simulink model "BMD_2_backup"  (R2025b)
settings: Solver=FixedStepAuto  StartTime=0.0  StopTime=15  FixedStep=0.005  RelTol=1e-3
values from neighbouring files (symbols this model uses):
  FPV_mass = 0.8    [Soft.m]
  g = 9.81    [Soft.m]
  ks = 0    [Soft.m]
  p_0 = 1013.25    [Soft.m]
  Q2Ts = forcetomotors()    [Soft.m]    (also in forcetomotors.m = inv(Ts2Q))
  takeOffDuration = 2    [Soft.m]
  Ts = 0.005    [Soft.m]
undefined symbols (not defined in the file or in its folder): CdA, DiscIntNeverNeededParam, Dw, kd_dz, kd_pos_dx, kd_pos_dy, kd_pq, kd_pr, kd_y, kd_z, ki_dz, ki_pos_dx, ki_pos_dy, ki_pq, ki_pr, ki_y, ki_z, kp_dz, kp_pos_dx, kp_pos_dy, kp_pos_x, kp_pos_y, kp_pq, kp_pr, kp_y, kp_z, pInitialization, rho
libraries: simulink x43, discretizing x18, slpidlib x3, SignalEditorBlockLib x2, shared6dof x1, dynamicsLibrary x1, aerolibasang x1, aerolibnav x1
(part 8 of 22)

== system BMD_2_backup/FCS/filters/Subsystem1/pitch_kalman ==
  ax,ay,az : Inport
  pitch : Inport  Port=2
  Atan2 : Trigonometry  Operator=atan2
  Compare To Constant : simulink/Logic and Bit Operations/Compare To Constant  relop=<=  const=8.5  OutDataTypeStr=boolean
  Compare To Constant1 : simulink/Logic and Bit Operations/Compare To Constant  relop=>=  const=11.5  OutDataTypeStr=boolean
  Data Type Conversion3 : DataTypeConversion  OutDataTypeStr=single  SaturateOnIntegerOverflow=off  RndMeth=Floor
  Demux : Demux  Outputs=3
  Gain1 : Gain  Gain=-1
  Kalman Filter1 : Subsystem  AncestorBlock=cstblocks/State Estimation/Kalman Filter  mask(ctrlKalmanFilter){TimeDomain=Discrete-Time, UseCurrentEstimator=on, ModelSource=Individual A, B, C, D matrices, ModelSourceVariable=ss(0.95,1,1,0,1), A=[1 -Ts;0 1], B=[Ts;0], C=[1 0], D=0, NumberOfStates=1, NumberOfInputs=1, NumberOfOutputs=1, InitialEstimateSource=Dialog, X0=[0; 0], P0=10, UseK=off, UseGH=off, NumberOfProcessNoiseInputs=1, G=1, TimeInvariantG=on, H=0, TimeInvariantH=on, Q=[0.001 0; 0 0.003], TimeInvariantQ=on, R=[1.0], TimeInvariantR=on, N=0, TimeInvariantN=on, AddInputPort=on, AddEnablePort=off, ExternalReset=None, OutputEstimatedY=off, OutputP=off, Ts=Ts}
      mask prompts: TimeDomain "Controllib:blocks:maskPromptKFTimeDomain"; UseCurrentEstimator "Controllib:blocks:maskPromptKFUseCurrentMeasurement"; ModelSource "Controllib:blocks:maskPromptKFModelSource"; ModelSourceVariable "Controllib:blocks:maskPromptKFModelSourceVariable"; A "Controllib:blocks:maskPromptKFA"; B "Controllib:blocks:maskPromptKFB"; C "Controllib:blocks:maskPromptKFC"; D "Controllib:blocks:maskPromptKFD"; NumberOfStates "Controllib:blocks:maskPromptKFNumberOfStates"; NumberOfInputs "Controllib:blocks:maskPromptKFNumberOfInputs"; NumberOfOutputs "Controllib:blocks:maskPromptKFNumberOfOutputs"; InitialEstimateSource "Controllib:blocks:maskPromptKFSource"; X0 "Controllib:blocks:maskPromptKFX0DT"; P0 "Controllib:blocks:maskPromptKFP0DT"; UseK "Controllib:blocks:maskPromptKFUseK"; UseGH "Controllib:blocks:maskPromptKFUseGH"; NumberOfProcessNoiseInputs "Controllib:blocks:maskPromptKFNumberOfProcessNoiseInputs"; G "Controllib:blocks:maskPromptKFG"; TimeInvariantG "Controllib:blocks:maskPromptKFTimeInvariantG"; H "Controllib:blocks:maskPromptKFH"; TimeInvariantH "Controllib:blocks:maskPromptKFTimeInvariantH"; Q "Controllib:blocks:maskPromptKFQ"; TimeInvariantQ "Controllib:blocks:maskPromptKFTimeInvariantQ"; R "Controllib:blocks:maskPromptKFR"; TimeInvariantR "Controllib:blocks:maskPromptKFTimeInvariantR"; N "Controllib:blocks:maskPromptKFN"; TimeInvariantN "Controllib:blocks:maskPromptKFTimeInvariantN"; AddInputPort "Controllib:blocks:maskPromptKFAddInputPort"; AddEnablePort "Controllib:blocks:maskPromptKFAddEnablePort"; ExternalReset "Simulink:blkprm_prompts:DelayBlkExternalReset"; OutputEstimatedY "Controllib:blocks:maskPromptKFOutputEstimatedY"; OutputP "Controllib:blocks:maskPromptKFOutputPZ"; Ts "Controllib:blocks:maskPromptKFTs"
      mask help: Controllib:blocks:maskPromptKFDescription
      mask init:
      | dlgParams.TimeDomain = TimeDomain;
      | dlgParams.UseCurrentEstimator = UseCurrentEstimator;
      | dlgParams.ModelSource = ModelSource;
      | dlgParams.ModelSourceVariable = ModelSourceVariable;
      | dlgParams.A = A;
      | dlgParams.B = B;
      | dlgParams.C = C;
      | dlgParams.D = D;
      | dlgParams.ModelHasFeedthrough = true();
      | dlgParams.NumberOfStates = NumberOfStates;
      | dlgParams.NumberOfInputs = NumberOfInputs;
      | dlgParams.NumberOfOutputs = NumberOfOutputs;
      | dlgParams.InitialEstimateSource = InitialEstimateSource;
      | dlgParams.X0 = X0;
      | dlgParams.P0 = P0;
      | dlgParams.UseGH = UseGH;
      | dlgParams.UseK = UseK;
      | dlgParams.NumberOfProcessNoiseInputs = NumberOfProcessNoiseInputs;
      | dlgParams.G = G;
      | dlgParams.TimeInvariantG = TimeInvariantG;
      | dlgParams.H = H;
      | dlgParams.TimeInvariantH = TimeInvariantH;
      | dlgParams.Q = Q;
      | dlgParams.TimeInvariantQ = TimeInvariantQ;
      | dlgParams.R = R;
      | dlgParams.TimeInvariantR = TimeInvariantR;
      | dlgParams.N = N;
      | dlgParams.TimeInvariantN = TimeInvariantN;
      | % Block options panel
      | dlgParams.OutputEstimatedY = OutputEstimatedY;
      | dlgParams.OutputP = OutputP;
      | dlgParams.AddEnablePort = AddEnablePort;
      | dlgParams.AddInputPort = AddInputPort;
      | dlgParams.ExternalReset = ExternalReset;
      | dlgParams.Ts = Ts;
      | [pInitialization,p] = ...
      |     controllib.internal.blocks.kalmanfilter.maskInitializationFcn(gcbh,dlgParams);
      | % Avoid storing dlg variables twice in the MaskWSVariables 
      | % block property
      | clear dlgParams;
      settings: LibrarySourceBlock=cstblocks/State Estimation/Kalman Filter
      mask Help: eval('controllib.internal.blocks.kalmanfilter.launchDocPage()')
      mask TypeOptions TimeDomain: Controllib:blocks:maskPromptKFTimeDomainDT | Controllib:blocks:maskPromptKFTimeDomainCT
      mask Callback TimeDomain: controllib.internal.blocks.kalmanfilter.dialogCallbacks(gcbh(),'comboBoxTimeDomain');
      mask Callback UseCurrentEstimator: controllib.internal.blocks.kalmanfilter.dialogCallbacks(gcbh(),'checkBoxUseCurrentEstimator');
      mask TypeOptions ModelSource: Controllib:blocks:maskPromptKFModelSourceLTIObject | Controllib:blocks:maskPromptKFModelSourceMatrices | Controllib:blocks:maskPromptKFSourceInport
      mask Callback ModelSource: controllib.internal.blocks.kalmanfilter.dialogCallbacks(gcbh(),'comboBoxModelSource');
      mask Callback ModelSourceVariable: controllib.internal.blocks.kalmanfilter.dialogCallbacks(gcbh(),'editBoxModelSourceVariable')
      mask TypeOptions InitialEstimateSource: Controllib:blocks:maskPromptKFSourceDialog | Controllib:blocks:maskPromptKFSourceInport
      mask Callback InitialEstimateSource: controllib.internal.blocks.kalmanfilter.dialogCallbacks(gcbh(),'comboBoxInitialEstimateSource');
      mask Callback UseK: controllib.internal.blocks.kalmanfilter.dialogCallbacks(gcbh(),'checkBoxUseK');
      mask Callback UseGH: controllib.internal.blocks.kalmanfilter.dialogCallbacks(gcbh(),'checkBoxUseGH');
      mask Callback TimeInvariantG: controllib.internal.blocks.kalmanfilter.dialogCallbacks(gcbh(),'checkBoxTimeInvariantGH');
      mask Callback TimeInvariantH: controllib.internal.blocks.kalmanfilter.dialogCallbacks(gcbh(),'checkBoxTimeInvariantGH');
      mask Callback TimeInvariantQ: controllib.internal.blocks.kalmanfilter.dialogCallbacks(gcbh(),'checkBoxTimeInvariantQRN');
      mask Callback TimeInvariantR: controllib.internal.blocks.kalmanfilter.dialogCallbacks(gcbh(),'checkBoxTimeInvariantQRN');
      mask Callback TimeInvariantN: controllib.internal.blocks.kalmanfilter.dialogCallbacks(gcbh(),'checkBoxTimeInvariantQRN');
      mask Callback AddInputPort: controllib.internal.blocks.kalmanfilter.dialogCallbacks(gcbh(),'checkBoxAddInputPort');
      mask TypeOptions ExternalReset: MemoryX/ExternalReset
      mask Callback OutputP: controllib.internal.blocks.kalmanfilter.dialogCallbacks(gcbh(),'checkBoxOutputP');
      mask DialogControl DescGroupVar Prompt: Controllib:blocks:maskPromptKFTitle
      mask DialogControl FilterSettingsContainer Prompt: Controllib:blocks:maskPromptKFContainerFilterSettings
      mask DialogControl TimeDomain Prompt: Time domain:
      mask DialogControl UseCurrentEstimator Prompt: Use the current measurement y[n] to improve xhat[n]
      mask DialogControl ModelParameterContainer Prompt: Controllib:blocks:maskPromptKFTabModelParameters
      mask DialogControl SystemModelContainer Prompt: Controllib:blocks:maskPromptKFContainerSystemModel
      mask DialogControl ModelSource Prompt: Model source:
      mask DialogControl ModelSourceVariable Prompt: Variable:
      mask DialogControl A Prompt: A:
      mask DialogControl B Prompt: B:
      mask DialogControl C Prompt: C:
      mask DialogControl D Prompt: D:
      mask DialogControl NumberOfStates Prompt: Number of states:
      mask DialogControl NumberOfInputs Prompt: Number of inputs:
      mask DialogControl NumberOfOutputs Prompt: Number of outputs:
      mask DialogControl InitialEstimatesContainer Prompt: Controllib:blocks:maskPromptKFContainerInitialEstimates
      mask DialogControl InitialEstimateSource Prompt: Source:
      mask DialogControl X0 Prompt: Initial states x[0]:
      mask DialogControl P0 Prompt: State estimation error covariance P[0]
      mask DialogControl NoiseCharacteristicsContainer Prompt: Controllib:blocks:maskPromptKFContainerNoiseCharacteristics
      mask DialogControl UseK Prompt: Use the Kalman Gain K from the model variable
      mask DialogControl UseGH Prompt: Use G and H matrices (default G=I and H=0)
      mask DialogControl NumberOfProcessNoiseInputs Prompt: Number of process noise inputs:
      mask DialogControl G Prompt: G:
      mask DialogControl TimeInvariantG Prompt: Time-invariant G
      mask DialogControl H Prompt: H:
      mask DialogControl TimeInvariantH Prompt: Time-invariant H
      mask DialogControl Q Prompt: Q:
      mask DialogControl TimeInvariantQ Prompt: Time-invariant Q
      mask DialogControl R Prompt: R:
      mask DialogControl TimeInvariantR Prompt: Time-invariant R
      mask DialogControl N Prompt: N:
      mask DialogControl TimeInvariantN Prompt: Time-invariant N
      mask DialogControl OptionsContainer Prompt: Controllib:blocks:maskPromptKFTabOptions
      mask DialogControl AdditionalInportsContainer Prompt: Controllib:blocks:maskPromptKFContainerAdditionalInports
      mask DialogControl AddInputPort Prompt: Add input port u
      mask DialogControl AddEnablePort Prompt: Add input port Enable to control measurement updates
      mask DialogControl ExternalReset Prompt: External reset:
      mask DialogControl AdditionalOutportsContainer Prompt: Controllib:blocks:maskPromptKFContainerAdditionalOutports
      mask DialogControl OutputEstimatedY Prompt: Output estimated model output y
      mask DialogControl OutputP Prompt: Output state estimation error covariance Z
      mask DialogControl Ts Prompt: Sample time (-1 for inherited):
  Kalman Filter2 : Subsystem  Commented=on  AncestorBlock=cstblocks/State Estimation/Kalman Filter  mask(ctrlKalmanFilter){TimeDomain=Discrete-Time, UseCurrentEstimator=on, ModelSource=Individual A, B, C, D matrices, ModelSourceVariable=ss(0.95,1,1,0,1), A=[1 0; 0 0], B=[Ts;0], C=[1 0], D=0, NumberOfStates=1, NumberOfInputs=1, NumberOfOutputs=1, InitialEstimateSource=Dialog, X0=[0; 0], P0=10, UseK=off, UseGH=off, NumberOfProcessNoiseInputs=1, G=1, TimeInvariantG=on, H=0, TimeInvariantH=on, Q=[1e-6 0; 0 0], TimeInvariantQ=on, R=100, TimeInvariantR=on, N=0, TimeInvariantN=on, AddInputPort=on, AddEnablePort=off, ExternalReset=None, OutputEstimatedY=off, OutputP=off, Ts=Ts}
      mask prompts: TimeDomain "Controllib:blocks:maskPromptKFTimeDomain"; UseCurrentEstimator "Controllib:blocks:maskPromptKFUseCurrentMeasurement"; ModelSource "Controllib:blocks:maskPromptKFModelSource"; ModelSourceVariable "Controllib:blocks:maskPromptKFModelSourceVariable"; A "Controllib:blocks:maskPromptKFA"; B "Controllib:blocks:maskPromptKFB"; C "Controllib:blocks:maskPromptKFC"; D "Controllib:blocks:maskPromptKFD"; NumberOfStates "Controllib:blocks:maskPromptKFNumberOfStates"; NumberOfInputs "Controllib:blocks:maskPromptKFNumberOfInputs"; NumberOfOutputs "Controllib:blocks:maskPromptKFNumberOfOutputs"; InitialEstimateSource "Controllib:blocks:maskPromptKFSource"; X0 "Controllib:blocks:maskPromptKFX0DT"; P0 "Controllib:blocks:maskPromptKFP0DT"; UseK "Controllib:blocks:maskPromptKFUseK"; UseGH "Controllib:blocks:maskPromptKFUseGH"; NumberOfProcessNoiseInputs "Controllib:blocks:maskPromptKFNumberOfProcessNoiseInputs"; G "Controllib:blocks:maskPromptKFG"; TimeInvariantG "Controllib:blocks:maskPromptKFTimeInvariantG"; H "Controllib:blocks:maskPromptKFH"; TimeInvariantH "Controllib:blocks:maskPromptKFTimeInvariantH"; Q "Controllib:blocks:maskPromptKFQ"; TimeInvariantQ "Controllib:blocks:maskPromptKFTimeInvariantQ"; R "Controllib:blocks:maskPromptKFR"; TimeInvariantR "Controllib:blocks:maskPromptKFTimeInvariantR"; N "Controllib:blocks:maskPromptKFN"; TimeInvariantN "Controllib:blocks:maskPromptKFTimeInvariantN"; AddInputPort "Controllib:blocks:maskPromptKFAddInputPort"; AddEnablePort "Controllib:blocks:maskPromptKFAddEnablePort"; ExternalReset "Simulink:blkprm_prompts:DelayBlkExternalReset"; OutputEstimatedY "Controllib:blocks:maskPromptKFOutputEstimatedY"; OutputP "Controllib:blocks:maskPromptKFOutputPZ"; Ts "Controllib:blocks:maskPromptKFTs"
      mask help: Controllib:blocks:maskPromptKFDescription
      mask init: same as BMD_2_backup/FCS/filters/Subsystem1/pitch_kalman/Kalman Filter1
      settings: LibrarySourceBlock=cstblocks/State Estimation/Kalman Filter
      mask Help: eval('controllib.internal.blocks.kalmanfilter.launchDocPage()')
      mask TypeOptions TimeDomain: Controllib:blocks:maskPromptKFTimeDomainDT | Controllib:blocks:maskPromptKFTimeDomainCT
      mask Callback TimeDomain: controllib.internal.blocks.kalmanfilter.dialogCallbacks(gcbh(),'comboBoxTimeDomain');
      mask Callback UseCurrentEstimator: controllib.internal.blocks.kalmanfilter.dialogCallbacks(gcbh(),'checkBoxUseCurrentEstimator');
      mask TypeOptions ModelSource: Controllib:blocks:maskPromptKFModelSourceLTIObject | Controllib:blocks:maskPromptKFModelSourceMatrices | Controllib:blocks:maskPromptKFSourceInport
      mask Callback ModelSource: controllib.internal.blocks.kalmanfilter.dialogCallbacks(gcbh(),'comboBoxModelSource');
      mask Callback ModelSourceVariable: controllib.internal.blocks.kalmanfilter.dialogCallbacks(gcbh(),'editBoxModelSourceVariable')
      mask TypeOptions InitialEstimateSource: Controllib:blocks:maskPromptKFSourceDialog | Controllib:blocks:maskPromptKFSourceInport
      mask Callback InitialEstimateSource: controllib.internal.blocks.kalmanfilter.dialogCallbacks(gcbh(),'comboBoxInitialEstimateSource');
      mask Callback UseK: controllib.internal.blocks.kalmanfilter.dialogCallbacks(gcbh(),'checkBoxUseK');
      mask Callback UseGH: controllib.internal.blocks.kalmanfilter.dialogCallbacks(gcbh(),'checkBoxUseGH');
      mask Callback TimeInvariantG: controllib.internal.blocks.kalmanfilter.dialogCallbacks(gcbh(),'checkBoxTimeInvariantGH');
      mask Callback TimeInvariantH: controllib.internal.blocks.kalmanfilter.dialogCallbacks(gcbh(),'checkBoxTimeInvariantGH');
      mask Callback TimeInvariantQ: controllib.internal.blocks.kalmanfilter.dialogCallbacks(gcbh(),'checkBoxTimeInvariantQRN');
      mask Callback TimeInvariantR: controllib.internal.blocks.kalmanfilter.dialogCallbacks(gcbh(),'checkBoxTimeInvariantQRN');
      mask Callback TimeInvariantN: controllib.internal.blocks.kalmanfilter.dialogCallbacks(gcbh(),'checkBoxTimeInvariantQRN');
      mask Callback AddInputPort: controllib.internal.blocks.kalmanfilter.dialogCallbacks(gcbh(),'checkBoxAddInputPort');
      mask TypeOptions ExternalReset: MemoryX/ExternalReset
      mask Callback OutputP: controllib.internal.blocks.kalmanfilter.dialogCallbacks(gcbh(),'checkBoxOutputP');
      mask DialogControl DescGroupVar Prompt: Controllib:blocks:maskPromptKFTitle
      mask DialogControl FilterSettingsContainer Prompt: Controllib:blocks:maskPromptKFContainerFilterSettings
      mask DialogControl TimeDomain Prompt: Time domain:
      mask DialogControl UseCurrentEstimator Prompt: Use the current measurement y[n] to improve xhat[n]
      mask DialogControl ModelParameterContainer Prompt: Controllib:blocks:maskPromptKFTabModelParameters
      mask DialogControl SystemModelContainer Prompt: Controllib:blocks:maskPromptKFContainerSystemModel
      mask DialogControl ModelSource Prompt: Model source:
      mask DialogControl ModelSourceVariable Prompt: Variable:
      mask DialogControl A Prompt: A:
      mask DialogControl B Prompt: B:
      mask DialogControl C Prompt: C:
      mask DialogControl D Prompt: D:
      mask DialogControl NumberOfStates Prompt: Number of states:
      mask DialogControl NumberOfInputs Prompt: Number of inputs:
      mask DialogControl NumberOfOutputs Prompt: Number of outputs:
      mask DialogControl InitialEstimatesContainer Prompt: Controllib:blocks:maskPromptKFContainerInitialEstimates
      mask DialogControl InitialEstimateSource Prompt: Source:
      mask DialogControl X0 Prompt: Initial states x[0]:
      mask DialogControl P0 Prompt: State estimation error covariance P[0]
      mask DialogControl NoiseCharacteristicsContainer Prompt: Controllib:blocks:maskPromptKFContainerNoiseCharacteristics
      mask DialogControl UseK Prompt: Use the Kalman Gain K from the model variable
      mask DialogControl UseGH Prompt: Use G and H matrices (default G=I and H=0)
      mask DialogControl NumberOfProcessNoiseInputs Prompt: Number of process noise inputs:
      mask DialogControl G Prompt: G:
      mask DialogControl TimeInvariantG Prompt: Time-invariant G
      mask DialogControl H Prompt: H:
      mask DialogControl TimeInvariantH Prompt: Time-invariant H
      mask DialogControl Q Prompt: Q:
      mask DialogControl TimeInvariantQ Prompt: Time-invariant Q
      mask DialogControl R Prompt: R:
      mask DialogControl TimeInvariantR Prompt: Time-invariant R
      mask DialogControl N Prompt: N:
      mask DialogControl TimeInvariantN Prompt: Time-invariant N
      mask DialogControl OptionsContainer Prompt: Controllib:blocks:maskPromptKFTabOptions
      mask DialogControl AdditionalInportsContainer Prompt: Controllib:blocks:maskPromptKFContainerAdditionalInports
      mask DialogControl AddInputPort Prompt: Add input port u
      mask DialogControl AddEnablePort Prompt: Add input port Enable to control measurement updates
      mask DialogControl ExternalReset Prompt: External reset:
      mask DialogControl AdditionalOutportsContainer Prompt: Controllib:blocks:maskPromptKFContainerAdditionalOutports
      mask DialogControl OutputEstimatedY Prompt: Output estimated model output y
      mask DialogControl OutputP Prompt: Output state estimation error covariance Z
      mask DialogControl Ts Prompt: Sample time (-1 for inherited):
  OR : Logic  Operator=NOR  IconShape=distinctive  AllPortsSameDT=off  OutDataTypeStr=boolean
  Rate Transition : RateTransition  OutPortSampleTime=Ts
  Rate Transition1 : RateTransition  OutPortSampleTime=Ts
  Rate Transition2 : RateTransition  OutPortSampleTime=Ts
  Scope : Scope
      settings: ActiveDisplayYMinimum=-1  ActiveDisplayYMaximum=1  DataLoggingVariableName=ScopeData43
  Selector1 : Selector  InputPortWidth=2  IndexOptions=Index vector (dialog)  Indices=1  OutputSizes=1
  Sqrt : Sqrt
  Sqrt1 : Sqrt
  Square{,1..4} (5 alike) : Math  Operator=square
  Sum : Sum  Inputs=++|
  Sum1 : Sum  Inputs=+|+|+
  Switch : Switch  Criteria=u2 > Threshold  SaturateOnIntegerOverflow=off  InputSameDT=off
  Unit Delay : UnitDelay  SampleTime=-1  HasFrameUpgradeWarning=on
  Out1 : Outport
  wires:
  ax,ay,az/1 -> Demux/1
  Selector1/1 -> Unit Delay/1, Rate Transition2/1
  Kalman Filter1/1(xhat) -> Selector1/1
  Rate Transition/1 -> Kalman Filter1/1(u)
  Rate Transition1/1 -> Kalman Filter1/2(y)
  Demux/3 -> Square4/1, Square1/1
  Demux/2 -> Square2/1, Square/1
  Square/1 -> Sum/1
  Square1/1 -> Sum/2
  Sum/1 -> Sqrt/1
  Sqrt/1 -> Atan2/2
  Demux/1 -> Square3/1, Gain1/1
  Data Type Conversion3/1 -> Out1/1
  Gain1/1 -> Atan2/1
  Atan2/1 -> Switch/1
  pitch/1 -> Rate Transition/1
  Sqrt1/1 -> Compare To Constant1/1, Compare To Constant/1
  Compare To Constant/1 -> OR/1
  Compare To Constant1/1 -> OR/2
  OR/1 -> Switch/2
  Unit Delay/1 -> Switch/3
  Switch/1 -> Rate Transition1/1
  Square3/1 -> Sum1/1
  Square2/1 -> Sum1/2
  Square4/1 -> Sum1/3
  Sum1/1 -> Sqrt1/1
  Rate Transition2/1 -> Scope/1, Data Type Conversion3/1

== system BMD_2_backup/FCS/filters/Subsystem1/roll_kalman ==
  ax,ay,az : Inport
  p : Inport  Port=2
  Atan2 : Trigonometry  Operator=atan2
  Compare To Constant : simulink/Logic and Bit Operations/Compare To Constant  relop=<=  const=8.5  OutDataTypeStr=boolean
  Compare To Constant1 : simulink/Logic and Bit Operations/Compare To Constant  relop=>=  const=11.5  OutDataTypeStr=boolean
  Data Type Conversion3 : DataTypeConversion  OutDataTypeStr=single  SaturateOnIntegerOverflow=off  RndMeth=Floor
  Demux : Demux  Outputs=3
  Kalman Filter2 : Subsystem  Commented=on  AncestorBlock=cstblocks/State Estimation/Kalman Filter  mask(ctrlKalmanFilter){TimeDomain=Discrete-Time, UseCurrentEstimator=on, ModelSource=Individual A, B, C, D matrices, ModelSourceVariable=ss(0.95,1,1,0,1), A=[1 0; 0 0], B=[Ts;0], C=[1 0], D=0, NumberOfStates=1, NumberOfInputs=1, NumberOfOutputs=1, InitialEstimateSource=Dialog, X0=[0; 0], P0=10, UseK=off, UseGH=off, NumberOfProcessNoiseInputs=1, G=1, TimeInvariantG=on, H=0, TimeInvariantH=on, Q=[1e-6 0; 0 0], TimeInvariantQ=on, R=100, TimeInvariantR=on, N=0, TimeInvariantN=on, AddInputPort=on, AddEnablePort=off, ExternalReset=None, OutputEstimatedY=off, OutputP=off, Ts=Ts}
      mask prompts: TimeDomain "Controllib:blocks:maskPromptKFTimeDomain"; UseCurrentEstimator "Controllib:blocks:maskPromptKFUseCurrentMeasurement"; ModelSource "Controllib:blocks:maskPromptKFModelSource"; ModelSourceVariable "Controllib:blocks:maskPromptKFModelSourceVariable"; A "Controllib:blocks:maskPromptKFA"; B "Controllib:blocks:maskPromptKFB"; C "Controllib:blocks:maskPromptKFC"; D "Controllib:blocks:maskPromptKFD"; NumberOfStates "Controllib:blocks:maskPromptKFNumberOfStates"; NumberOfInputs "Controllib:blocks:maskPromptKFNumberOfInputs"; NumberOfOutputs "Controllib:blocks:maskPromptKFNumberOfOutputs"; InitialEstimateSource "Controllib:blocks:maskPromptKFSource"; X0 "Controllib:blocks:maskPromptKFX0DT"; P0 "Controllib:blocks:maskPromptKFP0DT"; UseK "Controllib:blocks:maskPromptKFUseK"; UseGH "Controllib:blocks:maskPromptKFUseGH"; NumberOfProcessNoiseInputs "Controllib:blocks:maskPromptKFNumberOfProcessNoiseInputs"; G "Controllib:blocks:maskPromptKFG"; TimeInvariantG "Controllib:blocks:maskPromptKFTimeInvariantG"; H "Controllib:blocks:maskPromptKFH"; TimeInvariantH "Controllib:blocks:maskPromptKFTimeInvariantH"; Q "Controllib:blocks:maskPromptKFQ"; TimeInvariantQ "Controllib:blocks:maskPromptKFTimeInvariantQ"; R "Controllib:blocks:maskPromptKFR"; TimeInvariantR "Controllib:blocks:maskPromptKFTimeInvariantR"; N "Controllib:blocks:maskPromptKFN"; TimeInvariantN "Controllib:blocks:maskPromptKFTimeInvariantN"; AddInputPort "Controllib:blocks:maskPromptKFAddInputPort"; AddEnablePort "Controllib:blocks:maskPromptKFAddEnablePort"; ExternalReset "Simulink:blkprm_prompts:DelayBlkExternalReset"; OutputEstimatedY "Controllib:blocks:maskPromptKFOutputEstimatedY"; OutputP "Controllib:blocks:maskPromptKFOutputPZ"; Ts "Controllib:blocks:maskPromptKFTs"
      mask help: Controllib:blocks:maskPromptKFDescription
      mask init: same as BMD_2_backup/FCS/filters/Subsystem1/pitch_kalman/Kalman Filter1
      settings: LibrarySourceBlock=cstblocks/State Estimation/Kalman Filter
      mask Help: eval('controllib.internal.blocks.kalmanfilter.launchDocPage()')
      mask TypeOptions TimeDomain: Controllib:blocks:maskPromptKFTimeDomainDT | Controllib:blocks:maskPromptKFTimeDomainCT
      mask Callback TimeDomain: controllib.internal.blocks.kalmanfilter.dialogCallbacks(gcbh(),'comboBoxTimeDomain');
      mask Callback UseCurrentEstimator: controllib.internal.blocks.kalmanfilter.dialogCallbacks(gcbh(),'checkBoxUseCurrentEstimator');
      mask TypeOptions ModelSource: Controllib:blocks:maskPromptKFModelSourceLTIObject | Controllib:blocks:maskPromptKFModelSourceMatrices | Controllib:blocks:maskPromptKFSourceInport
      mask Callback ModelSource: controllib.internal.blocks.kalmanfilter.dialogCallbacks(gcbh(),'comboBoxModelSource');
      mask Callback ModelSourceVariable: controllib.internal.blocks.kalmanfilter.dialogCallbacks(gcbh(),'editBoxModelSourceVariable')
      mask TypeOptions InitialEstimateSource: Controllib:blocks:maskPromptKFSourceDialog | Controllib:blocks:maskPromptKFSourceInport
      mask Callback InitialEstimateSource: controllib.internal.blocks.kalmanfilter.dialogCallbacks(gcbh(),'comboBoxInitialEstimateSource');
      mask Callback UseK: controllib.internal.blocks.kalmanfilter.dialogCallbacks(gcbh(),'checkBoxUseK');
      mask Callback UseGH: controllib.internal.blocks.kalmanfilter.dialogCallbacks(gcbh(),'checkBoxUseGH');
      mask Callback TimeInvariantG: controllib.internal.blocks.kalmanfilter.dialogCallbacks(gcbh(),'checkBoxTimeInvariantGH');
      mask Callback TimeInvariantH: controllib.internal.blocks.kalmanfilter.dialogCallbacks(gcbh(),'checkBoxTimeInvariantGH');
      mask Callback TimeInvariantQ: controllib.internal.blocks.kalmanfilter.dialogCallbacks(gcbh(),'checkBoxTimeInvariantQRN');
      mask Callback TimeInvariantR: controllib.internal.blocks.kalmanfilter.dialogCallbacks(gcbh(),'checkBoxTimeInvariantQRN');
      mask Callback TimeInvariantN: controllib.internal.blocks.kalmanfilter.dialogCallbacks(gcbh(),'checkBoxTimeInvariantQRN');
      mask Callback AddInputPort: controllib.internal.blocks.kalmanfilter.dialogCallbacks(gcbh(),'checkBoxAddInputPort');
      mask TypeOptions ExternalReset: MemoryX/ExternalReset
      mask Callback OutputP: controllib.internal.blocks.kalmanfilter.dialogCallbacks(gcbh(),'checkBoxOutputP');
      mask DialogControl DescGroupVar Prompt: Controllib:blocks:maskPromptKFTitle
      mask DialogControl FilterSettingsContainer Prompt: Controllib:blocks:maskPromptKFContainerFilterSettings
      mask DialogControl TimeDomain Prompt: Time domain:
      mask DialogControl UseCurrentEstimator Prompt: Use the current measurement y[n] to improve xhat[n]
      mask DialogControl ModelParameterContainer Prompt: Controllib:blocks:maskPromptKFTabModelParameters
      mask DialogControl SystemModelContainer Prompt: Controllib:blocks:maskPromptKFContainerSystemModel
      mask DialogControl ModelSource Prompt: Model source:
      mask DialogControl ModelSourceVariable Prompt: Variable:
      mask DialogControl A Prompt: A:
      mask DialogControl B Prompt: B:
      mask DialogControl C Prompt: C:
      mask DialogControl D Prompt: D:
      mask DialogControl NumberOfStates Prompt: Number of states:
      mask DialogControl NumberOfInputs Prompt: Number of inputs:
      mask DialogControl NumberOfOutputs Prompt: Number of outputs:
      mask DialogControl InitialEstimatesContainer Prompt: Controllib:blocks:maskPromptKFContainerInitialEstimates
      mask DialogControl InitialEstimateSource Prompt: Source:
      mask DialogControl X0 Prompt: Initial states x[0]:
      mask DialogControl P0 Prompt: State estimation error covariance P[0]
      mask DialogControl NoiseCharacteristicsContainer Prompt: Controllib:blocks:maskPromptKFContainerNoiseCharacteristics
      mask DialogControl UseK Prompt: Use the Kalman Gain K from the model variable
      mask DialogControl UseGH Prompt: Use G and H matrices (default G=I and H=0)
      mask DialogControl NumberOfProcessNoiseInputs Prompt: Number of process noise inputs:
      mask DialogControl G Prompt: G:
      mask DialogControl TimeInvariantG Prompt: Time-invariant G
      mask DialogControl H Prompt: H:
      mask DialogControl TimeInvariantH Prompt: Time-invariant H
      mask DialogControl Q Prompt: Q:
      mask DialogControl TimeInvariantQ Prompt: Time-invariant Q
      mask DialogControl R Prompt: R:
      mask DialogControl TimeInvariantR Prompt: Time-invariant R
      mask DialogControl N Prompt: N:
      mask DialogControl TimeInvariantN Prompt: Time-invariant N
      mask DialogControl OptionsContainer Prompt: Controllib:blocks:maskPromptKFTabOptions
      mask DialogControl AdditionalInportsContainer Prompt: Controllib:blocks:maskPromptKFContainerAdditionalInports
      mask DialogControl AddInputPort Prompt: Add input port u
      mask DialogControl AddEnablePort Prompt: Add input port Enable to control measurement updates
      mask DialogControl ExternalReset Prompt: External reset:
      mask DialogControl AdditionalOutportsContainer Prompt: Controllib:blocks:maskPromptKFContainerAdditionalOutports
      mask DialogControl OutputEstimatedY Prompt: Output estimated model output y
      mask DialogControl OutputP Prompt: Output state estimation error covariance Z
      mask DialogControl Ts Prompt: Sample time (-1 for inherited):
  Kalman Filter3 : Subsystem  AncestorBlock=cstblocks/State Estimation/Kalman Filter  mask(ctrlKalmanFilter){TimeDomain=Discrete-Time, UseCurrentEstimator=on, ModelSource=Individual A, B, C, D matrices, ModelSourceVariable=ss(0.95,1,1,0,1), A=[1 -Ts;0 1], B=[Ts;0], C=[1 0], D=0, NumberOfStates=1, NumberOfInputs=1, NumberOfOutputs=1, InitialEstimateSource=Dialog, X0=[0; 0], P0=10, UseK=off, UseGH=off, NumberOfProcessNoiseInputs=1, G=1, TimeInvariantG=on, H=0, TimeInvariantH=on, Q=[0.001 0; 0 0.003], TimeInvariantQ=on, R=[1.0], TimeInvariantR=on, N=0, TimeInvariantN=on, AddInputPort=on, AddEnablePort=off, ExternalReset=None, OutputEstimatedY=off, OutputP=off, Ts=Ts}
      mask prompts: TimeDomain "Controllib:blocks:maskPromptKFTimeDomain"; UseCurrentEstimator "Controllib:blocks:maskPromptKFUseCurrentMeasurement"; ModelSource "Controllib:blocks:maskPromptKFModelSource"; ModelSourceVariable "Controllib:blocks:maskPromptKFModelSourceVariable"; A "Controllib:blocks:maskPromptKFA"; B "Controllib:blocks:maskPromptKFB"; C "Controllib:blocks:maskPromptKFC"; D "Controllib:blocks:maskPromptKFD"; NumberOfStates "Controllib:blocks:maskPromptKFNumberOfStates"; NumberOfInputs "Controllib:blocks:maskPromptKFNumberOfInputs"; NumberOfOutputs "Controllib:blocks:maskPromptKFNumberOfOutputs"; InitialEstimateSource "Controllib:blocks:maskPromptKFSource"; X0 "Controllib:blocks:maskPromptKFX0DT"; P0 "Controllib:blocks:maskPromptKFP0DT"; UseK "Controllib:blocks:maskPromptKFUseK"; UseGH "Controllib:blocks:maskPromptKFUseGH"; NumberOfProcessNoiseInputs "Controllib:blocks:maskPromptKFNumberOfProcessNoiseInputs"; G "Controllib:blocks:maskPromptKFG"; TimeInvariantG "Controllib:blocks:maskPromptKFTimeInvariantG"; H "Controllib:blocks:maskPromptKFH"; TimeInvariantH "Controllib:blocks:maskPromptKFTimeInvariantH"; Q "Controllib:blocks:maskPromptKFQ"; TimeInvariantQ "Controllib:blocks:maskPromptKFTimeInvariantQ"; R "Controllib:blocks:maskPromptKFR"; TimeInvariantR "Controllib:blocks:maskPromptKFTimeInvariantR"; N "Controllib:blocks:maskPromptKFN"; TimeInvariantN "Controllib:blocks:maskPromptKFTimeInvariantN"; AddInputPort "Controllib:blocks:maskPromptKFAddInputPort"; AddEnablePort "Controllib:blocks:maskPromptKFAddEnablePort"; ExternalReset "Simulink:blkprm_prompts:DelayBlkExternalReset"; OutputEstimatedY "Controllib:blocks:maskPromptKFOutputEstimatedY"; OutputP "Controllib:blocks:maskPromptKFOutputPZ"; Ts "Controllib:blocks:maskPromptKFTs"
      mask help: Controllib:blocks:maskPromptKFDescription
      mask init: same as BMD_2_backup/FCS/filters/Subsystem1/pitch_kalman/Kalman Filter1
      settings: LibrarySourceBlock=cstblocks/State Estimation/Kalman Filter
      mask Help: eval('controllib.internal.blocks.kalmanfilter.launchDocPage()')
      mask TypeOptions TimeDomain: Controllib:blocks:maskPromptKFTimeDomainDT | Controllib:blocks:maskPromptKFTimeDomainCT
      mask Callback TimeDomain: controllib.internal.blocks.kalmanfilter.dialogCallbacks(gcbh(),'comboBoxTimeDomain');
      mask Callback UseCurrentEstimator: controllib.internal.blocks.kalmanfilter.dialogCallbacks(gcbh(),'checkBoxUseCurrentEstimator');
      mask TypeOptions ModelSource: Controllib:blocks:maskPromptKFModelSourceLTIObject | Controllib:blocks:maskPromptKFModelSourceMatrices | Controllib:blocks:maskPromptKFSourceInport
      mask Callback ModelSource: controllib.internal.blocks.kalmanfilter.dialogCallbacks(gcbh(),'comboBoxModelSource');
      mask Callback ModelSourceVariable: controllib.internal.blocks.kalmanfilter.dialogCallbacks(gcbh(),'editBoxModelSourceVariable')
      mask TypeOptions InitialEstimateSource: Controllib:blocks:maskPromptKFSourceDialog | Controllib:blocks:maskPromptKFSourceInport
      mask Callback InitialEstimateSource: controllib.internal.blocks.kalmanfilter.dialogCallbacks(gcbh(),'comboBoxInitialEstimateSource');
      mask Callback UseK: controllib.internal.blocks.kalmanfilter.dialogCallbacks(gcbh(),'checkBoxUseK');
      mask Callback UseGH: controllib.internal.blocks.kalmanfilter.dialogCallbacks(gcbh(),'checkBoxUseGH');
      mask Callback TimeInvariantG: controllib.internal.blocks.kalmanfilter.dialogCallbacks(gcbh(),'checkBoxTimeInvariantGH');
      mask Callback TimeInvariantH: controllib.internal.blocks.kalmanfilter.dialogCallbacks(gcbh(),'checkBoxTimeInvariantGH');
      mask Callback TimeInvariantQ: controllib.internal.blocks.kalmanfilter.dialogCallbacks(gcbh(),'checkBoxTimeInvariantQRN');
      mask Callback TimeInvariantR: controllib.internal.blocks.kalmanfilter.dialogCallbacks(gcbh(),'checkBoxTimeInvariantQRN');
      mask Callback TimeInvariantN: controllib.internal.blocks.kalmanfilter.dialogCallbacks(gcbh(),'checkBoxTimeInvariantQRN');
      mask Callback AddInputPort: controllib.internal.blocks.kalmanfilter.dialogCallbacks(gcbh(),'checkBoxAddInputPort');
      mask TypeOptions ExternalReset: MemoryX/ExternalReset
      mask Callback OutputP: controllib.internal.blocks.kalmanfilter.dialogCallbacks(gcbh(),'checkBoxOutputP');
      mask DialogControl DescGroupVar Prompt: Controllib:blocks:maskPromptKFTitle
      mask DialogControl FilterSettingsContainer Prompt: Controllib:blocks:maskPromptKFContainerFilterSettings
      mask DialogControl TimeDomain Prompt: Time domain:
      mask DialogControl UseCurrentEstimator Prompt: Use the current measurement y[n] to improve xhat[n]
      mask DialogControl ModelParameterContainer Prompt: Controllib:blocks:maskPromptKFTabModelParameters
      mask DialogControl SystemModelContainer Prompt: Controllib:blocks:maskPromptKFContainerSystemModel
      mask DialogControl ModelSource Prompt: Model source:
      mask DialogControl ModelSourceVariable Prompt: Variable:
      mask DialogControl A Prompt: A:
      mask DialogControl B Prompt: B:
      mask DialogControl C Prompt: C:
      mask DialogControl D Prompt: D:
      mask DialogControl NumberOfStates Prompt: Number of states:
      mask DialogControl NumberOfInputs Prompt: Number of inputs:
      mask DialogControl NumberOfOutputs Prompt: Number of outputs:
      mask DialogControl InitialEstimatesContainer Prompt: Controllib:blocks:maskPromptKFContainerInitialEstimates
      mask DialogControl InitialEstimateSource Prompt: Source:
      mask DialogControl X0 Prompt: Initial states x[0]:
      mask DialogControl P0 Prompt: State estimation error covariance P[0]
      mask DialogControl NoiseCharacteristicsContainer Prompt: Controllib:blocks:maskPromptKFContainerNoiseCharacteristics
      mask DialogControl UseK Prompt: Use the Kalman Gain K from the model variable
      mask DialogControl UseGH Prompt: Use G and H matrices (default G=I and H=0)
      mask DialogControl NumberOfProcessNoiseInputs Prompt: Number of process noise inputs:
      mask DialogControl G Prompt: G:
      mask DialogControl TimeInvariantG Prompt: Time-invariant G
      mask DialogControl H Prompt: H:
      mask DialogControl TimeInvariantH Prompt: Time-invariant H
      mask DialogControl Q Prompt: Q:
      mask DialogControl TimeInvariantQ Prompt: Time-invariant Q
      mask DialogControl R Prompt: R:
      mask DialogControl TimeInvariantR Prompt: Time-invariant R
      mask DialogControl N Prompt: N:
      mask DialogControl TimeInvariantN Prompt: Time-invariant N
      mask DialogControl OptionsContainer Prompt: Controllib:blocks:maskPromptKFTabOptions
      mask DialogControl AdditionalInportsContainer Prompt: Controllib:blocks:maskPromptKFContainerAdditionalInports
      mask DialogControl AddInputPort Prompt: Add input port u
      mask DialogControl AddEnablePort Prompt: Add input port Enable to control measurement updates
      mask DialogControl ExternalReset Prompt: External reset:
      mask DialogControl AdditionalOutportsContainer Prompt: Controllib:blocks:maskPromptKFContainerAdditionalOutports
      mask DialogControl OutputEstimatedY Prompt: Output estimated model output y
      mask DialogControl OutputP Prompt: Output state estimation error covariance Z
      mask DialogControl Ts Prompt: Sample time (-1 for inherited):
  OR : Logic  Operator=NOR  IconShape=distinctive  AllPortsSameDT=off  OutDataTypeStr=boolean
  Rate Transition : RateTransition  OutPortSampleTime=Ts
  Rate Transition1 : RateTransition  OutPortSampleTime=Ts
  Rate Transition2 : RateTransition  OutPortSampleTime=Ts
  Scope : Scope
      settings: ActiveDisplayYMinimum=-22.571311950683594  ActiveDisplayYMaximum=40.743698120117188  DataLoggingVariableName=ScopeData47
  Selector : Selector  InputPortWidth=2  IndexOptions=Index vector (dialog)  Indices=1  OutputSizes=1
  Sqrt1 : Sqrt
  Square2 : Math  Operator=square
  Square3 : Math  Operator=square
  Square4 : Math  Operator=square
  Sum1 : Sum  Inputs=+|+|+
  Switch : Switch  Criteria=u2 > Threshold  SaturateOnIntegerOverflow=off  InputSameDT=off
  Unit Delay : UnitDelay  SampleTime=-1  HasFrameUpgradeWarning=on
  roll_f : Outport
  wires:
  ax,ay,az/1 -> Demux/1
  Demux/1 -> Square3/1
  Atan2/1 -> Switch/1
  p/1 -> Rate Transition/1
  Kalman Filter3/1(xhat) -> Selector/1
  Selector/1 -> Unit Delay/1, Rate Transition2/1
  Demux/2 -> Square2/1, Atan2/1
  Demux/3 -> Square4/1, Atan2/2
  Rate Transition/1 -> Kalman Filter3/1(u)
  Rate Transition1/1 -> Kalman Filter3/2(y)
  Square2/1 -> Sum1/2
  Square4/1 -> Sum1/3
  OR/1 -> Switch/2
  Sum1/1 -> Sqrt1/1
  Unit Delay/1 -> Switch/3
  Sqrt1/1 -> Compare To Constant1/1, Compare To Constant/1
  Square3/1 -> Sum1/1
  Compare To Constant1/1 -> OR/2
  Compare To Constant/1 -> OR/1
  Rate Transition2/1 -> Data Type Conversion3/1
  Switch/1 -> Rate Transition1/1
  Data Type Conversion3/1 -> Scope/1, roll_f/1

== system BMD_2_backup/FCS/filters/Subsystem1/yaw_filter ==
  note: This yaw estimate can drift with time.
  In1 : Inport
  Integrator1 : DiscreteIntegrator  SampleTime=0.005  OutDataTypeStr=single  ICPrevOutput=DiscIntNeverNeededParam  ICPrevScaledInput=DiscIntNeverNeededParam  mask(DiscretizedDiscreteIntegrator){}
      mask init:
      | %zoh
  Out1 : Outport
  wires:
  In1/1 -> Integrator1/1
  Integrator1/1 -> Out1/1

== system BMD_2_backup/Model/Subsystem/Motor Forces and Torques/For Each Subsystem ==
  Vb : Inport  PortDimensions=3
  rho : Inport  Port=2  PortDimensions=1
  Omega : Inport  Port=3
  w : Inport  Port=4  Partition=on  PartitionDimension=2  PartitionWidth=1  PartitionOffset=0
  D : Inport  Port=5  Partition=on  PartitionDimension=2  PartitionWidth=1  PartitionOffset=0
  For Each : ForEach  DisableCoverage=on
  Mux : Mux  Inputs=3
  Rotor Dynamics : dynamicsLibrary/Rotor Dynamics  SystemSampleTime=-1  VariantActivationTime=update diagram  EmptyChoice=off  PassThrough=off  PassThroughVariantControl=(default)  EmptyChoiceVariantControl=(default)  AllowFlexibleInterface=on  Latency=0  AutoFrameSizeCalculation=off
  Forces : Outport  ConcatenationDimension=2  VectorParamsAs1DForOutWhenUnconnected=off
  Moments : Outport  Port=2  ConcatenationDimension=2  VectorParamsAs1DForOutWhenUnconnected=off
  wires:
  Rotor Dynamics/1 -> Forces/1
  Rotor Dynamics/2 -> Moments/1
  Vb/1 -> Rotor Dynamics/1
  Omega/1 -> Rotor Dynamics/2
  rho/1 -> Rotor Dynamics/3
  D/1 -> Mux/3, Mux/1, Mux/2
  w/1 -> Rotor Dynamics/4
  Mux/1 -> Rotor Dynamics/5

== system BMD_2_backup/Model/Subsystem/Motor Forces and Torques/MotorsToW ==
  motors_datin : Inport
  Motordirections : Gain  Gain=[1 -1 1 -1]  ParamDataTypeStr=single  OutDataTypeStr=Inherit: Inherit via back propagation  SaturateOnIntegerOverflow=on
  Motordirections1 : Gain  Gain=[1 -1 1 -1]  ParamDataTypeStr=single  OutDataTypeStr=Inherit: Inherit via back propagation  SaturateOnIntegerOverflow=on
  Saturation5 : Saturate  UpperLimit=2047  LowerLimit=47  OutDataTypeStr=Inherit: Inherit via back propagation
  Scope : Scope  NumInputPorts=2
      settings: ActiveDisplayYMinimum=-37.836166415801024  ActiveDisplayYMaximum=37.836166415801024  DataLoggingVariableName=ScopeData72
  Signed Sqrt : Sqrt  Operator=signedSqrt  OutDataTypeStr=Inherit: Inherit via back propagation
  motorsToW2_Gain : Gain  Gain=[1 1 1 1]  ParamDataTypeStr=single  OutDataTypeStr=Inherit: Inherit via back propagation  SaturateOnIntegerOverflow=on
  omegas_datout : Outport  VectorParamsAs1DForOutWhenUnconnected=off
  wires:
  motorsToW2_Gain/1 -> Signed Sqrt/1
  Saturation5/1 -> Motordirections1/1
  Motordirections1/1 -> motorsToW2_Gain/1
  Signed Sqrt/1 -> Scope/2, omegas_datout/1
  motors_datin/1 -> Saturation5/1, Scope/1

== system BMD_2_backup/FCS/Controller/position_controller/pos_dx_pid/Anti-windup ==
  preSat : Inport  SampleTime=SampleTime
  postSat : Inport  Port=2  SampleTime=SampleTime
  P : Inport  Port=3  SampleTime=SampleTime
  preInt : Inport  Port=4  SampleTime=SampleTime
  Upper Limit : Inport  Port=5  SampleTime=SampleTime
  Lower Limit : Inport  Port=6  SampleTime=SampleTime
  Back Calculation : Subsystem  VariantControl=BackCalculation
  Cont. Clamping Ideal : Subsystem  VariantControl=ContClampingIdeal
  Cont. Clamping Parallel : Subsystem  VariantControl=ContClampingParallel
  Disabled : Subsystem  VariantControl=Disabled
  Disc. Clamping Ideal : Subsystem  VariantControl=DiscClampingIdeal
  Disc. Clamping Parallel : Subsystem  VariantControl=DiscClampingParallel
  Passthrough : Subsystem  VariantControl=Passthrough
  Out1 : Outport  SampleTime=SampleTime

== system BMD_2_backup/FCS/Controller/position_controller/pos_dx_pid/D Gain ==
  err : Inport  SampleTime=SampleTime
  D Gain : Inport  Port=2  SampleTime=SampleTime
  Disabled : Subsystem  VariantControl=Disabled
  External Parameters : Subsystem  VariantControl=ExternalParameters
  Internal Parameters : Subsystem  VariantControl=InternalParameters
  Out1 : Outport  SampleTime=SampleTime

== system BMD_2_backup/FCS/Controller/position_controller/pos_dx_pid/External Derivative ==
  err : Inport  SampleTime=SampleTime
  ydot : Inport  Port=2  SampleTime=SampleTime
  Disabled : Subsystem  VariantControl=Disabled
  Error : Subsystem  VariantControl=ErrorSignal
  External Ydot : Subsystem  VariantControl=ExternalYdot
  Out1 : Outport  SampleTime=SampleTime

== system BMD_2_backup/FCS/Controller/position_controller/pos_dx_pid/Filter ==
  Reset : Inport  SampleTime=SampleTime
  U : Inport  Port=2  SampleTime=SampleTime
  N : Inport  Port=3  SampleTime=SampleTime
  D0in : Inport  Port=4  SampleTime=SampleTime
  Nout : Inport  Port=5  SampleTime=SampleTime
  Ts : Inport  Port=6  SampleTime=SampleTime
  Cont. Filter : Subsystem  VariantControl=ContFilter
  Cont. Filter Only : Subsystem  VariantControl=ContFilterOnly
  Differentiator : Subsystem  VariantControl=Differentiator
  Disabled : Subsystem  VariantControl=Disabled
  Disc. Backward Euler Filter : Subsystem  VariantControl=BackwardEulerFilter
  Disc. Backward Euler Filter Only : Subsystem  VariantControl=BackwardEulerFilterOnly
  Disc. Forward Euler Filter : Subsystem  VariantControl=ForwardEulerFilter
  Disc. Forward Euler Filter Only : Subsystem  VariantControl=ForwardEulerFilterOnly
  Disc. Trapezoidal Filter : Subsystem  VariantControl=TrapezoidalFilter
  Disc. Trapezoidal Filter Only : Subsystem  VariantControl=TrapezoidalFilterOnly
  Passthrough : Subsystem  VariantControl=Passthrough
  Y : Outport  SampleTime=SampleTime

== system BMD_2_backup/FCS/Controller/position_controller/pos_dx_pid/Filter ICs ==
  D0 : Inport  SampleTime=SampleTime
  Disabled : Subsystem  VariantControl=Disabled
  External IC : Subsystem  VariantControl=ExternalICs
  Internal IC - Differentiator : Subsystem  VariantControl=InternalICsDifferentiator
  Internal IC - Filter : Subsystem  VariantControl=InternalICsFilter
  Out1 : Outport  SampleTime=SampleTime

== system BMD_2_backup/FCS/Controller/position_controller/pos_dx_pid/I Gain ==
  err : Inport  SampleTime=SampleTime
  I Gain : Inport  Port=2  SampleTime=SampleTime
  Disabled : Subsystem  VariantControl=Disabled
  External Parameters : Subsystem  VariantControl=ExternalParameters
  Internal Parameters : Subsystem  VariantControl=InternalParameters
  Out1 : Outport  SampleTime=SampleTime

== system BMD_2_backup/FCS/Controller/position_controller/pos_dx_pid/Ideal P Gain ==
  In1 : Inport  SampleTime=SampleTime
  P Gain : Inport  Port=2  SampleTime=SampleTime
  External Parameters : Subsystem  VariantControl=ExternalParameters
  Internal Parameters : Subsystem  VariantControl=InternalParameters
  Passthrough : Subsystem  VariantControl=Disabled
  Out1 : Outport  SampleTime=SampleTime

== system BMD_2_backup/FCS/Controller/position_controller/pos_dx_pid/Ideal P Gain Fdbk ==
  In1 : Inport  SampleTime=SampleTime
  P Gain : Inport  Port=2  SampleTime=SampleTime
  Disabled : Subsystem  VariantControl=Disabled
  External Parameters : Subsystem  VariantControl=ExternalParameters
  Internal Parameters : Subsystem  VariantControl=InternalParameters
  Passthrough : Subsystem  VariantControl=Passthrough
  Out1 : Outport  SampleTime=SampleTime

== system BMD_2_backup/FCS/Controller/position_controller/pos_dx_pid/Integrator ==
  U : Inport  SampleTime=SampleTime
  I0in : Inport  Port=2  SampleTime=SampleTime
  Reset : Inport  Port=3  SampleTime=SampleTime
  Continuous : Subsystem  VariantControl=Continuous
  Disabled : Subsystem  VariantControl=Disabled
  Discrete : Subsystem  VariantControl=Discrete
  state : Outport  SampleTime=SampleTime
  out : Outport  Port=2  SampleTime=SampleTime

== system BMD_2_backup/FCS/Controller/position_controller/pos_dx_pid/Integrator ICs ==
  I0 : Inport  SampleTime=SampleTime
  Disabled : Subsystem  VariantControl=Disabled
  External IC : Subsystem  VariantControl=ExternalICs
  Internal IC : Subsystem  VariantControl=InternalICs
  Out1 : Outport  SampleTime=SampleTime

== system BMD_2_backup/FCS/Controller/position_controller/pos_dx_pid/N Copy ==
  N Gain : Inport  SampleTime=SampleTime
  Disabled : Subsystem  VariantControl=Disabled
  Disabled wSignal Specification : Subsystem  VariantControl=Disabled_SignalSpec
  External Parameters : Subsystem  VariantControl=ExternalParameters
  Internal Parameters : Subsystem  VariantControl=InternalParameters
  Out1 : Outport  SampleTime=SampleTime

== system BMD_2_backup/FCS/Controller/position_controller/pos_dx_pid/N Gain ==
  U : Inport  SampleTime=SampleTime
  N Gain : Inport  Port=2  SampleTime=SampleTime
  Disabled : Subsystem  VariantControl=Disabled
  External Parameters : Subsystem  VariantControl=ExternalParameters
  Internal Parameters : Subsystem  VariantControl=InternalParameters
  Passthrough : Subsystem  VariantControl=Passthrough
  Out1 : Outport  SampleTime=SampleTime

== system BMD_2_backup/FCS/Controller/position_controller/pos_dx_pid/P Copy ==
  P Gain : Inport  SampleTime=SampleTime
  Disabled : Subsystem  VariantControl=Disabled
  External Parameters Ideal : Subsystem  VariantControl=ExternalParamsIdeal
  Internal Parameters Ideal : Subsystem  VariantControl=InternalParamsIdeal
  Out1 : Outport  SampleTime=SampleTime

== system BMD_2_backup/FCS/Controller/position_controller/pos_dx_pid/PID Compensator Formula ==

== system BMD_2_backup/FCS/Controller/position_controller/pos_dx_pid/Parallel P Gain ==
  err : Inport  SampleTime=SampleTime
  P Gain : Inport  Port=2  SampleTime=SampleTime
  Disabled : Subsystem  VariantControl=Disabled
  External Parameters : Subsystem  VariantControl=ExternalParameters
  Internal Parameters : Subsystem  VariantControl=InternalParameters
  Passthrough : Subsystem  VariantControl=Passthrough
  Out1 : Outport  SampleTime=SampleTime

== system BMD_2_backup/FCS/Controller/position_controller/pos_dx_pid/Reset Signal ==
  Reset : Inport  SampleTime=SampleTime
  Disabled : Subsystem  VariantControl=Disabled
  External Reset : Subsystem  VariantControl=ExternalReset
  Out1 : Outport  SampleTime=SampleTime

== system BMD_2_backup/FCS/Controller/position_controller/pos_dx_pid/Saturation ==
  In1 : Inport  SampleTime=SampleTime
  Upper Limit : Inport  Port=2  SampleTime=SampleTime
  Lower Limit : Inport  Port=3  SampleTime=SampleTime
  Enabled : Subsystem  VariantControl=Enabled
  External : Subsystem  VariantControl=External
  Passthrough : Subsystem  VariantControl=Disabled
  Out1 : Outport  SampleTime=SampleTime

== system BMD_2_backup/FCS/Controller/position_controller/pos_dx_pid/Saturation Fdbk ==
  In1 : Inport  SampleTime=SampleTime
  Upper Limit : Inport  Port=2  SampleTime=SampleTime
  Lower Limit : Inport  Port=3  SampleTime=SampleTime
  Disabled : Subsystem  VariantControl=Disabled
  Enabled : Subsystem  VariantControl=Enabled
  External : Subsystem  VariantControl=External
  Passthrough : Subsystem  VariantControl=Passthrough
  Out1 : Outport  SampleTime=SampleTime
